simulink library "qss_tb_library_aalto"  (Simulink 8.3)
settings: Solver=ode45  SolverMode=SingleTasking  StartTime=0.0  StopTime=1220  RelTol=1e-3
undefined symbols (not defined in the file): c_BT_E1, c_BT_E2, c_BT_E3, c_BT_E4, c_BT_L1, c_BT_L2, c_BT_L3, c_BT_L4, cap_BT, cc_done, delta_h_C_air, DiscIntNeverNeededParam, dw_GG_c, eff_FC_max, eta_EG_map, eta_EM_map, g, h, H_o_m, H_u, I_BT_max, i_FC_in, i_FC_max, k1, k2, k3, k4, k_cs, M_air, manual_gearbox, P_CVT_opt, power_max, Q_BT_0, Q_BT_IC, Q_BT_min, Q_SC_IC, r_wheel, rchg_map_BT, rdis_map_BT, rho, rho_f, soc_map_BT, t_c, T_CE_max, T_EG_c, T_EG_max, T_EM_max, T_z, U_BT_0, V, V_CE_map, V_FC_out, voc_map_BT, w_CE_max, w_CE_upper, w_CVT_opt, w_EG_row, w_EG_upper, w_EM_row, w_EM_upper ... (+1)
libraries: simulink x4
(part 3 of 4)

== system qss_tb_library_aalto/Controller/Gen-set Controller/Engine start control ==
  speed (m/s) : Inport
  soc : Inport  Port=2
  Constant11 : Constant  Value=10  OutDataTypeStr=double
  Cst_Q_BT_max : Constant  Value=soc_max
  Cst_Q_BT_min : Constant  Value=soc_min
  Data Type Conversion2 : DataTypeConversion  OutDataTypeStr=double
  Engine on off : Subsystem
  Hit Crossing : HitCross  HitCrossingOffset=0.5  HitCrossingDirection=rising
  Logical operator1 : Logic  Operator=OR
  Logical operator2 : Logic  Operator=OR
  Logical operator3 : Logic  Operator=OR
  Relational Operator : RelationalOperator  Operator=<=  OutDataTypeStr=boolean
  Relational Operator1 : RelationalOperator  OutDataTypeStr=boolean
  Terminator2 : Terminator
  low speed : simulink/Logic and Bit Operations/Compare To Constant  relop=<=  const=1  OutDataTypeStr=boolean
  speed min-max : Relay  OnSwitchValue=spd_max/3.6  OffSwitchValue=spd_min/3.6  OutDataTypeStr=Inherit: Inherit via back propagation
  tempo : Subsystem
      mask Display: disp('Tempo')
  engine on : Outport
  wires:
  Cst_Q_BT_min/1 -> Relational Operator/2
  Relational Operator/1 -> Logical operator3/2
  Cst_Q_BT_max/1 -> Relational Operator1/2
  speed (m/s)/1 -> speed min-max/1, low speed/1
  Logical operator3/1 -> Engine on off/1(S)
  Logical operator1/1 -> Engine on off/2(R)
  Engine on off/2(!Q) -> Terminator2/1
  soc/1 -> Relational Operator/1, Relational Operator1/1
  Relational Operator1/1 -> Logical operator1/2
  Constant11/1 -> tempo/2(time)
  Hit Crossing/1 -> tempo/1(flag)
  Engine on off/1(Q) -> Data Type Conversion2/1
  Data Type Conversion2/1 -> Hit Crossing/1, Logical operator2/1
  tempo/1(tempo) -> Logical operator2/2
  Logical operator2/1 -> engine on/1
  low speed/1 -> Logical operator1/1
  speed min-max/1 -> Logical operator3/1

== system qss_tb_library_aalto/Controller/Gen-set Controller/Power control ==
  power (W) : Inport
  speed (m/s) : Inport  Port=2
  soc : Inport  Port=3
  engine on : Inport  Port=4
  Constant5 : Constant  Value=0  OutDataTypeStr=double
  Constant6 : Constant  Value=0  OutDataTypeStr=double
  Cst_ctrl_speed*pi_30 : Constant  Value=ctrl_speed*pi/30  OutDataTypeStr=double  SampleTime=Inf
  Engine off : Mux  Inputs=2
  Engine on : Mux  Inputs=2
  Sum1 : Sum  SaturateOnIntegerOverflow=on  InputSameDT=on  OutDataTypeStr=Inherit: Same as first input
  Sum2 : Sum  SaturateOnIntegerOverflow=on  InputSameDT=on  OutDataTypeStr=Inherit: Same as first input
  Switch1 : Switch  Criteria=u2 > Threshold  Threshold=0.5  SaturateOnIntegerOverflow=on  InputSameDT=on
  charging power : Lookup_n-D  NumberOfTableDimensions=1  BreakpointsForDimension1=[0 0.6 0.71 0.75 0.8 1]  Table=[power_max power_max 0 0 -power_max/2 -power_max/2]  RndMeth=Simplest  InputSameDT=on
  power limit : Saturate  UpperLimit=power_max  LowerLimit=0
  speed correction : Lookup_n-D  NumberOfTableDimensions=1  BreakpointsForDimension1=[0 120]/3.6  Table=[0 spd_coeff]  RndMeth=Simplest  InputSameDT=on
  torque : Product  Inputs=*/  SaturateOnIntegerOverflow=on  RndMeth=Zero  InputSameDT=on  OutDataTypeStr=Inherit: Same as first input
  ctrl cmds : Outport
  wires:
  Constant5/1 -> Engine off/1
  Constant6/1 -> Engine off/2
  Engine on/1 -> Switch1/1
  Engine off/1 -> Switch1/3
  Sum1/1 -> power limit/1
  power limit/1 -> torque/1
  torque/1 -> Engine on/2
  Cst_ctrl_speed*pi_30/1 -> Engine on/1, torque/2
  engine on/1 -> Switch1/2
  Switch1/1 -> ctrl cmds/1
  speed (m/s)/1 -> speed correction/1
  soc/1 -> Sum2/1
  Sum2/1 -> charging power/1
  charging power/1 -> Sum1/2
  power (W)/1 -> Sum1/1
  speed correction/1 -> Sum2/2

== system qss_tb_library_aalto/Driving Cycle/Driving Cycle/Differentiation ==
  V_z : Inport
  Sum1 : Sum  Inputs=+-  SaturateOnIntegerOverflow=on  InputSameDT=on  OutDataTypeStr=Inherit: Same as first input
  Unit Delay1 : UnitDelay  SampleTime=h
  D_z : Outport  InitialOutput=0
  wires:
  Unit Delay1/1 -> Sum1/2
  V_z/1 -> Sum1/1, Unit Delay1/1
  Sum1/1 -> D_z/1

== system qss_tb_library_aalto/Driving Cycle/Driving Cycle/Integration ==
  V_z : Inport
  Gain4 : Gain  Gain=0.5*h  SaturateOnIntegerOverflow=on  OutDataTypeStr=Inherit: Same as input  ParamDataTypeStr=Inherit: Same as input
  Plant : UnitDelay  InitialCondition=1  SampleTime=h
  Sum2 : Sum  SaturateOnIntegerOverflow=on  InputSameDT=on  OutDataTypeStr=Inherit: Same as first input
  Sum4 : Sum  SaturateOnIntegerOverflow=on  InputSameDT=on  OutDataTypeStr=Inherit: Same as first input
  Unit Delay2 : UnitDelay  SampleTime=h
  x_tot : Outport  InitialOutput=0
  wires:
  Sum2/1 -> Gain4/1
  Unit Delay2/1 -> Sum2/2
  V_z/1 -> Sum2/1, Unit Delay2/1
  Gain4/1 -> Sum4/2
  Sum4/1 -> Plant/1
  Plant/1 -> Sum4/1, x_tot/1

== system qss_tb_library_aalto/Driving Cycle/Driving Cycle v2/Differentiation ==
  V_z : Inport
  Sum1 : Sum  Inputs=+-  SaturateOnIntegerOverflow=on  InputSameDT=on  OutDataTypeStr=Inherit: Same as first input
  Unit Delay1 : UnitDelay  SampleTime=h
  D_z : Outport  InitialOutput=0
  wires:
  Sum1/1 -> D_z/1
  V_z/1 -> Unit Delay1/1, Sum1/1
  Unit Delay1/1 -> Sum1/2

== system qss_tb_library_aalto/Driving Cycle/Driving Cycle v2/Integration ==
  V_z : Inport
  Gain4 : Gain  Gain=0.5*h  SaturateOnIntegerOverflow=on  OutDataTypeStr=Inherit: Same as input  ParamDataTypeStr=Inherit: Same as input
  Plant : UnitDelay  InitialCondition=1  SampleTime=h
  Sum2 : Sum  SaturateOnIntegerOverflow=on  InputSameDT=on  OutDataTypeStr=Inherit: Same as first input
  Sum4 : Sum  SaturateOnIntegerOverflow=on  InputSameDT=on  OutDataTypeStr=Inherit: Same as first input
  Unit Delay2 : UnitDelay  SampleTime=h
  x_tot : Outport  InitialOutput=0
  wires:
  Plant/1 -> x_tot/1, Sum4/1
  Sum4/1 -> Plant/1
  Gain4/1 -> Sum4/2
  V_z/1 -> Unit Delay2/1, Sum2/1
  Unit Delay2/1 -> Sum2/2
  Sum2/1 -> Gain4/1

== system qss_tb_library_aalto/Driving Cycle/Driving Cycle v3/Differentiation ==
  V_z : Inport
  Sum1 : Sum  Inputs=+-  SaturateOnIntegerOverflow=on  InputSameDT=on  OutDataTypeStr=Inherit: Same as first input
  Unit Delay1 : UnitDelay  SampleTime=h
  D_z : Outport  InitialOutput=0
  wires:
  Unit Delay1/1 -> Sum1/2
  V_z/1 -> Sum1/1, Unit Delay1/1
  Sum1/1 -> D_z/1

== system qss_tb_library_aalto/Driving Cycle/Driving Cycle v3/Integration ==
  V_z : Inport
  Gain4 : Gain  Gain=0.5*h  SaturateOnIntegerOverflow=on  OutDataTypeStr=Inherit: Same as input  ParamDataTypeStr=Inherit: Same as input
  Plant : UnitDelay  InitialCondition=1  SampleTime=h
  Sum2 : Sum  SaturateOnIntegerOverflow=on  InputSameDT=on  OutDataTypeStr=Inherit: Same as first input
  Sum4 : Sum  SaturateOnIntegerOverflow=on  InputSameDT=on  OutDataTypeStr=Inherit: Same as first input
  Unit Delay2 : UnitDelay  SampleTime=h
  x_tot : Outport  InitialOutput=0
  wires:
  Sum2/1 -> Gain4/1
  Unit Delay2/1 -> Sum2/2
  V_z/1 -> Sum2/1, Unit Delay2/1
  Gain4/1 -> Sum4/2
  Sum4/1 -> Plant/1
  Plant/1 -> Sum4/1, x_tot/1

== system qss_tb_library_aalto/Energy Buffer/Battery/Battery voltage ==
  Q_BT : Inport
  P_BT : Inport  Port=2
  Charging : Subsystem
  Discharging : Subsystem
  Enable charging : Subsystem
  Enable discharging : Subsystem
  Enable idle : Subsystem
  Idle : Subsystem
  Product : Product  Inputs=/*  SaturateOnIntegerOverflow=on  RndMeth=Zero  InputSameDT=on  OutDataTypeStr=Inherit: Same as first input
  Supervision battery : Subsystem
  Switch : Switch  Threshold=0.5  SaturateOnIntegerOverflow=on  InputSameDT=on
  Switch1 : Switch  Threshold=0.5  SaturateOnIntegerOverflow=on  InputSameDT=on
  U_BT : Outport  InitialOutput=0
  I_BT : Outport  Port=2  InitialOutput=0
  wires:
  Enable idle/1(e_Z) -> Idle/Enable
  Charging/1(U_BT_L) -> Switch/1
  Switch1/1 -> Switch/3
  Idle/1(U_BT_E) -> Switch1/3
  Discharging/1(U_BT_E) -> Switch1/1
  P_BT/1 -> Charging/2(P_BT), Enable charging/1(P_BT), Enable idle/1(P_BT), Product/2, Discharging/2(P_BT), Enable discharging/1(P_BT)
  Enable discharging/1(e_E) -> Discharging/Enable, Switch1/2
  Product/1 -> Supervision battery/3(I_BT), I_BT/1
  Q_BT/1 -> Supervision battery/1(Q_BT), Charging/1(Q_BT), Discharging/1(Q_BT), Idle/1(Q_BT)
  Enable charging/1(e_E) -> Charging/Enable, Switch/2
  Switch/1 -> Product/1, Supervision battery/2(U_BT), U_BT/1

== system qss_tb_library_aalto/Energy Buffer/Battery v2/cell model ==
  current : Inport
  soc calculation : Subsystem
  voltage calculation : Subsystem
  voltage_out : Outport
  voc_out : Outport  Port=2
  rint_out : Outport  Port=3
  soc_out : Outport  Port=4
  wires:
  current/1 -> voltage calculation/2(Current), soc calculation/1(current)
  voltage calculation/3(Rint) -> rint_out/1
  voltage calculation/1(Voc) -> voc_out/1
  voltage calculation/2(voltage) -> voltage_out/1
  soc calculation/1(soc) -> voltage calculation/1(SOC (prev)), soc_out/1

== system qss_tb_library_aalto/Energy Buffer/Battery v3/cell model ==
  current : Inport
  Switch1 : Switch  SaturateOnIntegerOverflow=on  InputSameDT=on
  coulombic efficiency : Gain  Gain=0.99
  soc calculation : Subsystem
  voltage calculation : Subsystem
  voltage_out : Outport
  voc_out : Outport  Port=2
  rint_out : Outport  Port=3
  soc_out : Outport  Port=4
  wires:
  soc calculation/1(soc) -> soc_out/1, voltage calculation/1(SOC (prev))
  voltage calculation/2(voltage) -> voltage_out/1
  voltage calculation/1(Voc) -> voc_out/1
  voltage calculation/3(Rint) -> rint_out/1
  coulombic efficiency/1 -> Switch1/3
  current/1 -> coulombic efficiency/1, Switch1/1, Switch1/2
  Switch1/1 -> voltage calculation/2(Current), soc calculation/1(current)

== system qss_tb_library_aalto/Energy Buffer/Supercapacitor/Supervision supercap ==
  Q_SC : Inport
  P_SC : Inport  Port=2
  Charge: P > 0 : Gain  Gain=4*C_SC^2*R_SC  SaturateOnIntegerOverflow=on  OutDataTypeStr=Inherit: Same as input  ParamDataTypeStr=Inherit: Same as input
  Constant6 : Constant  Value=U_SC_max
  Constant7 : Constant  Value=P_SC_max
  Gain : Gain  Gain=1/C_SC  SaturateOnIntegerOverflow=on  OutDataTypeStr=Inherit: Same as input  ParamDataTypeStr=Inherit: Same as input
  Math Function : Math  Operator=square  SaturateOnIntegerOverflow=on
  Saturation1 : Saturate  UpperLimit=0  LowerLimit=-inf
  Saturation2 : Saturate  UpperLimit=0  LowerLimit=-inf
  Saturation3 : Saturate  UpperLimit=0  LowerLimit=-inf
  Stop Simulation : Stop
  Stop Simulation1 : Stop
  Stop Simulation2 : Stop
  Sum1 : Sum  Inputs=-+  SaturateOnIntegerOverflow=on  InputSameDT=on  OutDataTypeStr=Inherit: Same as first input
  Sum2 : Sum  Inputs=+-  SaturateOnIntegerOverflow=on  InputSameDT=on  OutDataTypeStr=Inherit: Same as first input
  Sum4 : Sum  SaturateOnIntegerOverflow=on  InputSameDT=on  OutDataTypeStr=Inherit: Same as first input
  wires:
  Math Function/1 -> Sum2/1
  Q_SC/1 -> Math Function/1, Gain/1
  Constant7/1 -> Sum4/2
  Constant6/1 -> Sum1/2
  Sum4/1 -> Saturation3/1
  Sum2/1 -> Saturation2/1
  Gain/1 -> Sum1/1
  Sum1/1 -> Saturation1/1
  Charge: P > 0/1 -> Sum2/2
  P_SC/1 -> Charge: P > 0/1, Sum4/1
  Saturation1/1 -> Stop Simulation/1
  Saturation2/1 -> Stop Simulation1/1
  Saturation3/1 -> Stop Simulation2/1

== system qss_tb_library_aalto/Energy Buffer/Supercapacitor v2/Supervision supercap ==
  Q_SC : Inport
  P_SC : Inport  Port=2
  Charge: P > 0 : Gain  Gain=4*C_SC^2*R_SC  SaturateOnIntegerOverflow=on  OutDataTypeStr=Inherit: Same as input  ParamDataTypeStr=Inherit: Same as input
  Constant6 : Constant  Value=U_SC_max
  Constant7 : Constant  Value=P_SC_max
  Gain : Gain  Gain=1/C_SC  SaturateOnIntegerOverflow=on  OutDataTypeStr=Inherit: Same as input  ParamDataTypeStr=Inherit: Same as input
  Math Function : Math  Operator=square  SaturateOnIntegerOverflow=on
  Saturation1 : Saturate  UpperLimit=0  LowerLimit=-inf
  Saturation2 : Saturate  UpperLimit=0  LowerLimit=-inf
  Saturation3 : Saturate  UpperLimit=0  LowerLimit=-inf
  Stop Simulation : Stop
  Stop Simulation1 : Stop
  Stop Simulation2 : Stop
  Sum1 : Sum  Inputs=-+  SaturateOnIntegerOverflow=on  InputSameDT=on  OutDataTypeStr=Inherit: Same as first input
  Sum2 : Sum  Inputs=+-  SaturateOnIntegerOverflow=on  InputSameDT=on  OutDataTypeStr=Inherit: Same as first input
  Sum4 : Sum  SaturateOnIntegerOverflow=on  InputSameDT=on  OutDataTypeStr=Inherit: Same as first input
  wires:
  Saturation3/1 -> Stop Simulation2/1
  Saturation2/1 -> Stop Simulation1/1
  Saturation1/1 -> Stop Simulation/1
  P_SC/1 -> Sum4/1, Charge: P > 0/1
  Charge: P > 0/1 -> Sum2/2
  Sum1/1 -> Saturation1/1
  Gain/1 -> Sum1/1
  Sum2/1 -> Saturation2/1
  Sum4/1 -> Saturation3/1
  Constant6/1 -> Sum1/2
  Constant7/1 -> Sum4/2
  Q_SC/1 -> Gain/1, Math Function/1
  Math Function/1 -> Sum2/1

== system qss_tb_library_aalto/Energy Buffer/Supercapacitor v3/Supervision supercap ==
  Q_SC : Inport
  P_SC : Inport  Port=2
  Charge: P > 0 : Gain  Gain=4*C_SC^2*R_SC  SaturateOnIntegerOverflow=on  OutDataTypeStr=Inherit: Same as input  ParamDataTypeStr=Inherit: Same as input
  Constant6 : Constant  Value=U_SC_max
  Constant7 : Constant  Value=P_SC_max
  Gain : Gain  Gain=1/C_SC  SaturateOnIntegerOverflow=on  OutDataTypeStr=Inherit: Same as input  ParamDataTypeStr=Inherit: Same as input
  Math Function : Math  Operator=square  SaturateOnIntegerOverflow=on
  Saturation1 : Saturate  UpperLimit=0  LowerLimit=-inf
  Saturation2 : Saturate  UpperLimit=0  LowerLimit=-inf
  Saturation3 : Saturate  UpperLimit=0  LowerLimit=-inf
  Stop Simulation : Stop
  Stop Simulation1 : Stop
  Stop Simulation2 : Stop
  Sum1 : Sum  Inputs=-+  SaturateOnIntegerOverflow=on  InputSameDT=on  OutDataTypeStr=Inherit: Same as first input
  Sum2 : Sum  Inputs=+-  SaturateOnIntegerOverflow=on  InputSameDT=on  OutDataTypeStr=Inherit: Same as first input
  Sum4 : Sum  SaturateOnIntegerOverflow=on  InputSameDT=on  OutDataTypeStr=Inherit: Same as first input
  wires:
  Math Function/1 -> Sum2/1
  Q_SC/1 -> Math Function/1, Gain/1
  Constant7/1 -> Sum4/2
  Constant6/1 -> Sum1/2
  Sum4/1 -> Saturation3/1
  Sum2/1 -> Saturation2/1
  Gain/1 -> Sum1/1
  Sum1/1 -> Saturation1/1
  Charge: P > 0/1 -> Sum2/2
  P_SC/1 -> Charge: P > 0/1, Sum4/1
  Saturation1/1 -> Stop Simulation/1
  Saturation2/1 -> Stop Simulation1/1
  Saturation3/1 -> Stop Simulation2/1

== system qss_tb_library_aalto/Energy Converter/Combustion Engine (Willans-approximation)/Detect fuel cutoff ==
  P_CE_fuel : Inport
  T_CE : Inport  Port=2
  Constant1 : Constant  Value=ENABLE_FUEL_CUTOFF
  Constant3 : Constant  Value=P_CE_cutoff
  Decision : Switch  Threshold=0.5
  Detect fuel cutoff : Switch  Threshold=T_CE_cutoff + 0.01  SaturateOnIntegerOverflow=on  InputSameDT=on
  P_CE : Outport
  wires:
  Decision/1 -> P_CE/1
  Constant1/1 -> Decision/2
  Detect fuel cutoff/1 -> Decision/1
  P_CE_fuel/1 -> Decision/3, Detect fuel cutoff/1
  T_CE/1 -> Detect fuel cutoff/2
  Constant3/1 -> Detect fuel cutoff/3

== system qss_tb_library_aalto/Energy Converter/Combustion Engine (Willans-approximation)/Detect idle ==
  P_CE_fuel : Inport
  w_CE : Inport  Port=2
  T_CE : Inport  Port=3
  Constant3 : Constant  Value=P_CE_idle
  Idle detection : Fcn  Expr=(u(1) <= w_CE_idle) * (u(2) <= T_CE_idle)
  Mux : Mux  Inputs=2
  Switch2 : Switch  Threshold=0.5  SaturateOnIntegerOverflow=on  InputSameDT=on
  P_CE : Outport  InitialOutput=0
  wires:
  Constant3/1 -> Switch2/1
  Switch2/1 -> P_CE/1
  P_CE_fuel/1 -> Switch2/3
  Idle detection/1 -> Switch2/2
  w_CE/1 -> Mux/1
  T_CE/1 -> Mux/2
  Mux/1 -> Idle detection/1

== system qss_tb_library_aalto/Energy Converter/Combustion Engine (Willans-approximation)/Engine efficiency ==
  w_CE : Inport
  T_CE : Inport  Port=2
  Constant3 : Constant  Value=p_me0g
  Product1 : Product  Inputs=*/  SaturateOnIntegerOverflow=on  RndMeth=Zero  InputSameDT=on  OutDataTypeStr=Inherit: Same as first input
  Sum : Sum  SaturateOnIntegerOverflow=on  InputSameDT=on  OutDataTypeStr=Inherit: Same as first input
  p_me : Fcn  Expr=4*pi*u/V_d
  p_me0 : Sum  SaturateOnIntegerOverflow=on  InputSameDT=on  OutDataTypeStr=Inherit: Same as first input
  p_mef : Fcn  Expr=k1 * (k2 + k3*(S^2)*(u^2)) * PI * sqrt(k4/B)
  p_mf : Fcn  Expr=u/e
  eta_CE : Outport  InitialOutput=0
  wires:
  Product1/1 -> eta_CE/1
  p_me/1 -> Sum/1, Product1/1
  Sum/1 -> p_mf/1
  p_mf/1 -> Product1/2
  p_me0/1 -> Sum/2
  T_CE/1 -> p_me/1
  w_CE/1 -> p_mef/1
  p_mef/1 -> p_me0/1
  Constant3/1 -> p_me0/2

== system qss_tb_library_aalto/Energy Converter/Combustion Engine (consumption map)/Detect fuel cutoff ==
  P_CE_fuel : Inport
  T_CE : Inport  Port=2
  Constant1 : Constant  Value=ENABLE_FUEL_CUTOFF
  Constant3 : Constant  Value=P_CE_cutoff
  Decision : Switch  Threshold=0.5
  Detect fuel cutoff : Switch  Threshold=T_CE_cutoff + 0.01  SaturateOnIntegerOverflow=on  InputSameDT=on
  P_CE : Outport
  wires:
  Constant3/1 -> Detect fuel cutoff/3
  T_CE/1 -> Detect fuel cutoff/2
  P_CE_fuel/1 -> Detect fuel cutoff/1, Decision/3
  Detect fuel cutoff/1 -> Decision/1
  Constant1/1 -> Decision/2
  Decision/1 -> P_CE/1

== system qss_tb_library_aalto/Energy Converter/Combustion Engine (consumption map)/Detect idle ==
  P_CE_fuel : Inport
  w_CE : Inport  Port=2
  T_CE : Inport  Port=3
  Constant3 : Constant  Value=P_CE_idle
  Idle detection : Fcn  Expr=(u(1) <= w_CE_idle) * (u(2) <= T_CE_idle)
  Mux : Mux  Inputs=2
  Switch2 : Switch  Threshold=0.5  SaturateOnIntegerOverflow=on  InputSameDT=on
  P_CE : Outport  InitialOutput=0
  wires:
  Mux/1 -> Idle detection/1
  T_CE/1 -> Mux/2
  w_CE/1 -> Mux/1
  Idle detection/1 -> Switch2/2
  P_CE_fuel/1 -> Switch2/3
  Switch2/1 -> P_CE/1
  Constant3/1 -> Switch2/1

== system qss_tb_library_aalto/Energy Converter/Combustion Engine (consumption map)/Detect overload and overspeed ==
  w_CE : Inport
  T_CE : Inport  Port=2
  Abs : Abs  SaturateOnIntegerOverflow=on
  Constant : Constant  Value=w_CE_upper
  Maximum torque : Lookup  InputValues=w_CE_max  Table=T_CE_max  SaturateOnIntegerOverflow=on
  Saturation : Saturate  UpperLimit=0  LowerLimit=-inf
  Saturation1 : Saturate  UpperLimit=0  LowerLimit=-inf
  Stop Simulation : Stop
  Stop Simulation1 : Stop
  Sum : Sum  Inputs=+-  SaturateOnIntegerOverflow=on  InputSameDT=on  OutDataTypeStr=Inherit: Same as first input
  Sum1 : Sum  Inputs=+-  SaturateOnIntegerOverflow=on  InputSameDT=on  OutDataTypeStr=Inherit: Same as first input
  wires:
  Sum/1 -> Saturation/1
  w_CE/1 -> Maximum torque/1, Sum1/2
  T_CE/1 -> Abs/1
  Maximum torque/1 -> Sum/1
  Abs/1 -> Sum/2
  Saturation/1 -> Stop Simulation/1
  Constant/1 -> Sum1/1
  Sum1/1 -> Saturation1/1
  Saturation1/1 -> Stop Simulation1/1

== system qss_tb_library_aalto/Energy Converter/Combustion Engine (hybrid vehicle)/Detect fuel cutoff ==
  P_CE_fuel : Inport
  T_CE : Inport  Port=2
  Constant1 : Constant  Value=ENABLE_FUEL_CUTOFF
  Constant3 : Constant  Value=P_CE_cutoff
  Decision : Switch  Threshold=0.5
  Detect fuel cutoff : Switch  Threshold=T_CE_cutoff + 0.01  SaturateOnIntegerOverflow=on  InputSameDT=on
  P_CE : Outport
  wires:
  Decision/1 -> P_CE/1
  Constant1/1 -> Decision/2
  Detect fuel cutoff/1 -> Decision/1
  P_CE_fuel/1 -> Decision/3, Detect fuel cutoff/1
  T_CE/1 -> Detect fuel cutoff/2
  Constant3/1 -> Detect fuel cutoff/3

== system qss_tb_library_aalto/Energy Converter/Combustion Engine (hybrid vehicle)/Detect idle ==
  P_CE_fuel : Inport
  w_CE : Inport  Port=2
  T_CE : Inport  Port=3
  Constant3 : Constant  Value=P_CE_idle
  Idle detection : Fcn  Expr=(u(1) <= w_CE_idle) * (u(2) <= T_CE_idle)
  Mux : Mux  Inputs=2
  Switch2 : Switch  Threshold=0.5  SaturateOnIntegerOverflow=on  InputSameDT=on
  P_CE : Outport  InitialOutput=0
  wires:
  Constant3/1 -> Switch2/1
  Switch2/1 -> P_CE/1
  P_CE_fuel/1 -> Switch2/3
  Idle detection/1 -> Switch2/2
  w_CE/1 -> Mux/1
  T_CE/1 -> Mux/2
  Mux/1 -> Idle detection/1

== system qss_tb_library_aalto/Energy Converter/Combustion Engine (hybrid vehicle)/Detect overload and overspeed ==
  w_CE : Inport
  T_CE : Inport  Port=2
  Abs : Abs  SaturateOnIntegerOverflow=on
  Constant : Constant  Value=w_CE_upper
  Maximum torque : Lookup  InputValues=w_CE_max  Table=T_CE_max  SaturateOnIntegerOverflow=on
  Saturation : Saturate  UpperLimit=0  LowerLimit=-inf
  Saturation1 : Saturate  UpperLimit=0  LowerLimit=-inf
  Stop Simulation : Stop
  Stop Simulation1 : Stop
  Sum : Sum  Inputs=+-  SaturateOnIntegerOverflow=on  InputSameDT=on  OutDataTypeStr=Inherit: Same as first input
  Sum1 : Sum  Inputs=+-  SaturateOnIntegerOverflow=on  InputSameDT=on  OutDataTypeStr=Inherit: Same as first input
  wires:
  Saturation1/1 -> Stop Simulation1/1
  Sum1/1 -> Saturation1/1
  Constant/1 -> Sum1/1
  Saturation/1 -> Stop Simulation/1
  Abs/1 -> Sum/2
  Maximum torque/1 -> Sum/1
  T_CE/1 -> Abs/1
  w_CE/1 -> Sum1/2, Maximum torque/1
  Sum/1 -> Saturation/1

== system qss_tb_library_aalto/Energy Converter/Combustion Engine (hybrid vehicle)/torque limit ==
  w : Inport
  T : Inport  Port=2
  Constant2 : Constant  Value=T_CE_cutoff
  Maximum torque : Lookup  InputValues=w_CE_max  Table=T_CE_max  SaturateOnIntegerOverflow=on
  saturation with inputs : Subsystem
  T_lim : Outport
  wires:
  Maximum torque/1 -> saturation with inputs/1(upper limit in)
  Constant2/1 -> saturation with inputs/3(lower limit in)
  w/1 -> Maximum torque/1
  T/1 -> saturation with inputs/2(signal in)
  saturation with inputs/1(signal out) -> T_lim/1

== system qss_tb_library_aalto/Energy Converter/Combustion Engine (hybrid vehicle) v2/Detect fuel cutoff ==
  P_CE_fuel : Inport
  T_ctrl : Inport  Port=2
  Constant1 : Constant  Value=ENABLE_FUEL_CUTOFF
  Constant3 : Constant  Value=P_CE_cutoff
  Decision : Switch  Threshold=0.5
  Detect fuel cutoff : Switch  SaturateOnIntegerOverflow=on  InputSameDT=on
  P_CE : Outport
  wires:
  Constant3/1 -> Detect fuel cutoff/3
  T_ctrl/1 -> Detect fuel cutoff/2
  P_CE_fuel/1 -> Detect fuel cutoff/1, Decision/3
  Detect fuel cutoff/1 -> Decision/1
  Constant1/1 -> Decision/2
  Decision/1 -> P_CE/1

== system qss_tb_library_aalto/Energy Converter/Combustion Engine (hybrid vehicle) v2/Detect idle ==
  w_CE : Inport
  T_in : Inport  Port=2
  Constant1 : Constant  Value=P_aux
  Constant11 : Constant  Value=0  OutDataTypeStr=double
  Constant2 : Constant  Value=w_CE_idle
  Constant3 : Constant  Value=P_CE_idle
  Idle detection : Fcn  Expr=(u(2) <= T_CE_idle)
  Mux : Mux  Inputs=2
  Power : Sum  SaturateOnIntegerOverflow=on  InputSameDT=on  OutDataTypeStr=Inherit: Same as first input
  Product : Product  SaturateOnIntegerOverflow=on  RndMeth=Zero  InputSameDT=on  OutDataTypeStr=Inherit: Same as first input
  Product1 : Product  Inputs=*/  SaturateOnIntegerOverflow=on  RndMeth=Zero  InputSameDT=on  OutDataTypeStr=Inherit: Same as first input
  Rate Limiter : RateLimiter  RisingSlewLimit=100  FallingSlewLimit=-250
  Switch1 : Switch  Criteria=u2 > Threshold  SaturateOnIntegerOverflow=on  InputSameDT=on
  Switch2 : Switch  Threshold=0.5  SaturateOnIntegerOverflow=on  InputSameDT=on
  Switch3 : Switch  Threshold=0.5  SaturateOnIntegerOverflow=on  InputSameDT=on
  w_out : Outport  InitialOutput=0
  T_out : Outport  Port=2  InitialOutput=0
  wires:
  Mux/1 -> Idle detection/1
  T_in/1 -> Product/1, Mux/2
  w_CE/1 -> Switch3/3, Product/2, Mux/1
  Idle detection/1 -> Switch3/2, Switch2/2
  Constant3/1 -> Switch2/1
  Constant1/1 -> Power/2
  Switch2/1 -> Power/1
  Product/1 -> Switch2/3
  Power/1 -> Product1/1
  Product1/1 -> Switch1/1
  Switch1/1 -> T_out/1
  Constant11/1 -> Switch1/3
  Constant2/1 -> Switch3/1
  Switch3/1 -> Rate Limiter/1
  Rate Limiter/1 -> Switch1/2, w_out/1, Product1/2

== system qss_tb_library_aalto/Energy Converter/Combustion Engine (hybrid vehicle) v2/Detect overload and overspeed ==
  w_CE : Inport
  T_CE : Inport  Port=2
  Abs : Abs  SaturateOnIntegerOverflow=on
  Constant : Constant  Value=w_CE_upper
  Maximum torque : Lookup  InputValues=w_CE_max  Table=T_CE_max  SaturateOnIntegerOverflow=on
  Saturation : Saturate  UpperLimit=0  LowerLimit=-inf
  Saturation1 : Saturate  UpperLimit=0  LowerLimit=-inf
  Stop Simulation : Stop
  Stop Simulation1 : Stop
  Sum : Sum  Inputs=+-  SaturateOnIntegerOverflow=on  InputSameDT=on  OutDataTypeStr=Inherit: Same as first input
  Sum1 : Sum  Inputs=+-  SaturateOnIntegerOverflow=on  InputSameDT=on  OutDataTypeStr=Inherit: Same as first input
  wires:
  Sum/1 -> Saturation/1
  w_CE/1 -> Maximum torque/1, Sum1/2
  T_CE/1 -> Abs/1
  Maximum torque/1 -> Sum/1
  Abs/1 -> Sum/2
  Saturation/1 -> Stop Simulation/1
  Constant/1 -> Sum1/1
  Sum1/1 -> Saturation1/1
  Saturation1/1 -> Stop Simulation1/1

== system qss_tb_library_aalto/Energy Converter/Combustion Engine (hybrid vehicle) v2/torque limit ==
  w : Inport
  T : Inport  Port=2
  Constant2 : Constant  Value=T_CE_cutoff
  Maximum torque : Lookup  InputValues=w_CE_max  Table=T_CE_max  SaturateOnIntegerOverflow=on
  saturation with inputs : Subsystem
  T_lim : Outport
  wires:
  saturation with inputs/1(signal out) -> T_lim/1
  T/1 -> saturation with inputs/2(signal in)
  w/1 -> Maximum torque/1
  Constant2/1 -> saturation with inputs/3(lower limit in)
  Maximum torque/1 -> saturation with inputs/1(upper limit in)

== system qss_tb_library_aalto/Energy Converter/Combustion Engine v2/Detect fuel cutoff ==
  P_CE_fuel : Inport
  T_CE : Inport  Port=2
  Constant1 : Constant  Value=ENABLE_FUEL_CUTOFF
  Constant3 : Constant  Value=P_CE_cutoff
  Decision : Switch  Threshold=0.5
  Detect fuel cutoff : Switch  Threshold=T_CE_cutoff + 0.01  SaturateOnIntegerOverflow=on  InputSameDT=on
  P_CE : Outport
  wires:
  Decision/1 -> P_CE/1
  Constant1/1 -> Decision/2
  Detect fuel cutoff/1 -> Decision/1
  P_CE_fuel/1 -> Decision/3, Detect fuel cutoff/1
  T_CE/1 -> Detect fuel cutoff/2
  Constant3/1 -> Detect fuel cutoff/3

== system qss_tb_library_aalto/Energy Converter/Combustion Engine v2/Detect idle ==
  P_CE_fuel : Inport
  w_CE : Inport  Port=2
  T_CE : Inport  Port=3
  Constant3 : Constant  Value=P_CE_idle
  Idle detection : Fcn  Expr=(u(1) <= w_CE_idle) * (u(2) <= T_CE_idle)
  Mux : Mux  Inputs=2
  Switch2 : Switch  Threshold=0.5  SaturateOnIntegerOverflow=on  InputSameDT=on
  P_CE : Outport  InitialOutput=0
  wires:
  Constant3/1 -> Switch2/1
  Switch2/1 -> P_CE/1
  P_CE_fuel/1 -> Switch2/3
  Idle detection/1 -> Switch2/2
  w_CE/1 -> Mux/1
  T_CE/1 -> Mux/2
  Mux/1 -> Idle detection/1

== system qss_tb_library_aalto/Energy Converter/Combustion Engine v2/Detect overload and overspeed ==
  w_CE : Inport
  T_CE : Inport  Port=2
  Abs : Abs  SaturateOnIntegerOverflow=on
  Constant : Constant  Value=w_CE_upper
  Maximum torque : Lookup  InputValues=w_CE_max  Table=T_CE_max  SaturateOnIntegerOverflow=on
  Saturation : Saturate  UpperLimit=0  LowerLimit=-inf
  Saturation1 : Saturate  UpperLimit=0  LowerLimit=-inf
  Stop Simulation : Stop
  Stop Simulation1 : Stop
  Sum : Sum  Inputs=+-  SaturateOnIntegerOverflow=on  InputSameDT=on  OutDataTypeStr=Inherit: Same as first input
  Sum1 : Sum  Inputs=+-  SaturateOnIntegerOverflow=on  InputSameDT=on  OutDataTypeStr=Inherit: Same as first input
  wires:
  Saturation1/1 -> Stop Simulation1/1
  Sum1/1 -> Saturation1/1
  Constant/1 -> Sum1/1
  Saturation/1 -> Stop Simulation/1
  Abs/1 -> Sum/2
  Maximum torque/1 -> Sum/1
  T_CE/1 -> Abs/1
  w_CE/1 -> Sum1/2, Maximum torque/1
  Sum/1 -> Saturation/1

== system qss_tb_library_aalto/Energy Converter/Combustion Engine v3/Detect fuel cutoff ==
  P_CE_fuel : Inport
  T_gear : Inport  Port=2
  Constant1 : Constant  Value=ENABLE_FUEL_CUTOFF
  Constant3 : Constant  Value=P_CE_cutoff
  Decision : Switch  Threshold=0.5
  Detect fuel cutoff : Switch  SaturateOnIntegerOverflow=on  InputSameDT=on
  P_CE : Outport
  wires:
  Constant3/1 -> Detect fuel cutoff/3
  T_gear/1 -> Detect fuel cutoff/2
  P_CE_fuel/1 -> Detect fuel cutoff/1, Decision/3
  Detect fuel cutoff/1 -> Decision/1
  Constant1/1 -> Decision/2
  Decision/1 -> P_CE/1

== system qss_tb_library_aalto/Energy Converter/Combustion Engine v3/Detect idle ==
  w_CE : Inport
  T_in : Inport  Port=2
  Constant1 : Constant  Value=P_aux
  Constant11 : Constant  Value=0  OutDataTypeStr=double
  Constant3 : Constant  Value=P_CE_idle
  Idle detection : Fcn  Expr=(u(1) <= w_CE_idle) * (u(2) <= T_CE_idle)
  Mux : Mux  Inputs=2
  Power : Sum  SaturateOnIntegerOverflow=on  InputSameDT=on  OutDataTypeStr=Inherit: Same as first input
  Product : Product  SaturateOnIntegerOverflow=on  RndMeth=Zero  InputSameDT=on  OutDataTypeStr=Inherit: Same as first input
  Product1 : Product  Inputs=*/  SaturateOnIntegerOverflow=on  RndMeth=Zero  InputSameDT=on  OutDataTypeStr=Inherit: Same as first input
  Switch1 : Switch  Criteria=u2 > Threshold  SaturateOnIntegerOverflow=on  InputSameDT=on
  Switch2 : Switch  Threshold=0.5  SaturateOnIntegerOverflow=on  InputSameDT=on
  T_out : Outport  InitialOutput=0
  wires:
  Mux/1 -> Idle detection/1
  T_in/1 -> Product/1, Mux/2
  w_CE/1 -> Switch1/2, Product1/2, Product/2, Mux/1
  Idle detection/1 -> Switch2/2
  Constant3/1 -> Switch2/1
  Constant1/1 -> Power/2
  Switch2/1 -> Power/1
  Product/1 -> Switch2/3
  Power/1 -> Product1/1
  Constant11/1 -> Switch1/3
  Product1/1 -> Switch1/1
  Switch1/1 -> T_out/1

== system qss_tb_library_aalto/Energy Converter/Combustion Engine v3/Detect overload and overspeed ==
  w_CE : Inport
  T_CE : Inport  Port=2
  Abs : Abs  SaturateOnIntegerOverflow=on
  Constant : Constant  Value=w_CE_upper
  Maximum torque : Lookup  InputValues=w_CE_max  Table=T_CE_max  SaturateOnIntegerOverflow=on
  Saturation : Saturate  UpperLimit=0  LowerLimit=-inf
  Saturation1 : Saturate  UpperLimit=0  LowerLimit=-inf
  Stop Simulation : Stop
  Stop Simulation1 : Stop
  Sum : Sum  Inputs=+-  SaturateOnIntegerOverflow=on  InputSameDT=on  OutDataTypeStr=Inherit: Same as first input
  Sum1 : Sum  Inputs=+-  SaturateOnIntegerOverflow=on  InputSameDT=on  OutDataTypeStr=Inherit: Same as first input
  wires:
  Sum/1 -> Saturation/1
  w_CE/1 -> Maximum torque/1, Sum1/2
  T_CE/1 -> Abs/1
  Maximum torque/1 -> Sum/1
  Abs/1 -> Sum/2
  Saturation/1 -> Stop Simulation/1
  Constant/1 -> Sum1/1
  Sum1/1 -> Saturation1/1
  Saturation1/1 -> Stop Simulation1/1

== system qss_tb_library_aalto/Energy Converter/Electric Generator/Detect overload and overspeed ==
  w_EG : Inport
  T_EG : Inport  Port=2
  Abs : Abs  SaturateOnIntegerOverflow=on
  Constant : Constant  Value=w_EG_upper
  Maximum torque : Lookup  InputValues=w_EG_row  Table=T_EG_max  SaturateOnIntegerOverflow=on
  Saturation : Saturate  UpperLimit=0  LowerLimit=-inf
  Saturation1 : Saturate  UpperLimit=0  LowerLimit=-inf
  Stop Simulation : Stop
  Stop Simulation1 : Stop
  Sum : Sum  Inputs=+-  SaturateOnIntegerOverflow=on  InputSameDT=on  OutDataTypeStr=Inherit: Same as first input
  Sum1 : Sum  Inputs=+-  SaturateOnIntegerOverflow=on  InputSameDT=on  OutDataTypeStr=Inherit: Same as first input
  wires:
  Sum/1 -> Saturation/1
  w_EG/1 -> Maximum torque/1, Sum1/2
  T_EG/1 -> Abs/1
  Maximum torque/1 -> Sum/1
  Abs/1 -> Sum/2
  Saturation/1 -> Stop Simulation/1
  Constant/1 -> Sum1/1
  Sum1/1 -> Saturation1/1
  Saturation1/1 -> Stop Simulation1/1

== system qss_tb_library_aalto/Energy Converter/Electric Generator v2/Detect overload and overspeed ==
  w_EG : Inport
  T_EG : Inport  Port=2
  Abs : Abs  SaturateOnIntegerOverflow=on
  Constant : Constant  Value=w_EG_upper
  Maximum torque : Lookup  InputValues=w_EG_row  Table=T_EG_max  SaturateOnIntegerOverflow=on
  Saturation : Saturate  UpperLimit=0  LowerLimit=-inf
  Saturation1 : Saturate  UpperLimit=0  LowerLimit=-inf
  Stop Simulation : Stop
  Stop Simulation1 : Stop
  Sum : Sum  Inputs=+-  SaturateOnIntegerOverflow=on  InputSameDT=on  OutDataTypeStr=Inherit: Same as first input
  Sum1 : Sum  Inputs=+-  SaturateOnIntegerOverflow=on  InputSameDT=on  OutDataTypeStr=Inherit: Same as first input
  wires:
  Saturation1/1 -> Stop Simulation1/1
  Sum1/1 -> Saturation1/1
  Constant/1 -> Sum1/1
  Saturation/1 -> Stop Simulation/1
  Abs/1 -> Sum/2
  Maximum torque/1 -> Sum/1
  T_EG/1 -> Abs/1
  w_EG/1 -> Sum1/2, Maximum torque/1
  Sum/1 -> Saturation/1

== system qss_tb_library_aalto/Energy Converter/Electric Generator v3/Detect overload and overspeed ==
  w_EG : Inport
  T_EG : Inport  Port=2
  Abs : Abs  SaturateOnIntegerOverflow=on
  Constant : Constant  Value=w_EG_upper
  Maximum torque : Lookup  InputValues=w_EG_row  Table=T_EG_max  SaturateOnIntegerOverflow=on
  Saturation : Saturate  UpperLimit=0  LowerLimit=-inf
  Saturation1 : Saturate  UpperLimit=0  LowerLimit=-inf
  Stop Simulation : Stop
  Stop Simulation1 : Stop
  Sum : Sum  Inputs=+-  SaturateOnIntegerOverflow=on  InputSameDT=on  OutDataTypeStr=Inherit: Same as first input
  Sum1 : Sum  Inputs=+-  SaturateOnIntegerOverflow=on  InputSameDT=on  OutDataTypeStr=Inherit: Same as first input
  wires:
  Saturation1/1 -> Stop Simulation1/1
  Sum1/1 -> Saturation1/1
  Constant/1 -> Sum1/1
  Saturation/1 -> Stop Simulation/1
  Abs/1 -> Sum/2
  Maximum torque/1 -> Sum/1
  T_EG/1 -> Abs/1
  w_EG/1 -> Sum1/2, Maximum torque/1
  Sum/1 -> Saturation/1

== system qss_tb_library_aalto/Energy Converter/Electric Motor/Detect overload and overspeed ==
  w_EM : Inport
  T_EM : Inport  Port=2
  Abs : Abs  SaturateOnIntegerOverflow=on
  Constant : Constant  Value=w_EM_upper
  Maximum torque : Lookup  InputValues=w_EM_row  Table=T_EM_max  SaturateOnIntegerOverflow=on
  Saturation : Saturate  UpperLimit=0  LowerLimit=-inf
  Saturation1 : Saturate  UpperLimit=0  LowerLimit=-inf
  Stop Simulation : Stop
  Stop Simulation1 : Stop
  Sum : Sum  Inputs=+-  SaturateOnIntegerOverflow=on  InputSameDT=on  OutDataTypeStr=Inherit: Same as first input
  Sum1 : Sum  Inputs=+-  SaturateOnIntegerOverflow=on  InputSameDT=on  OutDataTypeStr=Inherit: Same as first input
  wires:
  Saturation1/1 -> Stop Simulation1/1
  Sum1/1 -> Saturation1/1
  Constant/1 -> Sum1/1
  Saturation/1 -> Stop Simulation/1
  Abs/1 -> Sum/2
  Maximum torque/1 -> Sum/1
  T_EM/1 -> Abs/1
  w_EM/1 -> Sum1/2, Maximum torque/1
  Sum/1 -> Saturation/1

== system qss_tb_library_aalto/Energy Converter/Electric Motor v2/Detect overload and overspeed ==
  w_EM : Inport
  T_EM : Inport  Port=2
  Abs : Abs  SaturateOnIntegerOverflow=on
  Constant : Constant  Value=w_EM_upper
  Maximum torque : Lookup  InputValues=w_EM_row  Table=T_EM_max*over_factor  SaturateOnIntegerOverflow=on
  Saturation : Saturate  UpperLimit=0  LowerLimit=-inf
  Saturation1 : Saturate  UpperLimit=0  LowerLimit=-inf
  Stop Simulation : Stop
  Stop Simulation1 : Stop
  Sum : Sum  Inputs=+-  SaturateOnIntegerOverflow=on  InputSameDT=on  OutDataTypeStr=Inherit: Same as first input
  Sum1 : Sum  Inputs=+-  SaturateOnIntegerOverflow=on  InputSameDT=on  OutDataTypeStr=Inherit: Same as first input
  wires:
  Sum/1 -> Saturation/1
  w_EM/1 -> Maximum torque/1, Sum1/2
  T_EM/1 -> Abs/1
  Maximum torque/1 -> Sum/1
  Abs/1 -> Sum/2
  Saturation/1 -> Stop Simulation/1
  Constant/1 -> Sum1/1
  Sum1/1 -> Saturation1/1
  Saturation1/1 -> Stop Simulation1/1

== system qss_tb_library_aalto/Energy Converter/Fuel Cell/Compressor with E-motor ==
  note: Air mass flow
  P_FC : Inport
  1/2 O2 for 1 H2 : Gain  Gain=1/2  SaturateOnIntegerOverflow=on  OutDataTypeStr=Inherit: Same as input  ParamDataTypeStr=Inherit: Same as input
  Air enthalpy : Gain  Gain=delta_h_C_air  SaturateOnIntegerOverflow=on  OutDataTypeStr=Inherit: Same as input  ParamDataTypeStr=Inherit: Same as input
  Air to fuel ratio : Gain  Gain=l_air  SaturateOnIntegerOverflow=on  OutDataTypeStr=Inherit: Same as input  ParamDataTypeStr=Inherit: Same as input
  E-motor efficiency : Gain  Gain=1/eta_EM_C  SaturateOnIntegerOverflow=on  OutDataTypeStr=Inherit: Same as input  ParamDataTypeStr=Inherit: Same as input
  Inverse O2  fraction : Gain  Gain=100/21  SaturateOnIntegerOverflow=on  OutDataTypeStr=Inherit: Same as input  ParamDataTypeStr=Inherit: Same as input
  Lower heating value : Gain  Gain=1/H_o_m  SaturateOnIntegerOverflow=on  OutDataTypeStr=Inherit: Same as input  ParamDataTypeStr=Inherit: Same as input
  Molecular weight : Gain  Gain=M_air  SaturateOnIntegerOverflow=on  OutDataTypeStr=Inherit: Same as input  ParamDataTypeStr=Inherit: Same as input
  To Workspace4 : ToWorkspace  VariableName=P_EM_C  SampleTime=1
  Unit Delay : UnitDelay  SampleTime=h
  P_EM_C : Outport  InitialOutput=0
  wires:
  Air enthalpy/1 -> E-motor efficiency/1
  Air to fuel ratio/1 -> Air enthalpy/1
  Unit Delay/1 -> Lower heating value/1
  Molecular weight/1 -> Air to fuel ratio/1
  Lower heating value/1 -> 1/2 O2 for 1 H2/1
  1/2 O2 for 1 H2/1 -> Inverse O2  fraction/1
  Inverse O2  fraction/1 -> Molecular weight/1
  E-motor efficiency/1 -> P_EM_C/1, To Workspace4/1
  P_FC/1 -> Unit Delay/1

== system qss_tb_library_aalto/Energy Converter/Fuel Cell/Supervision of current density ==
  "   i_FC" : Inport
  Constant6 : Constant  Value=i_FC_max
  Saturation1 : Saturate  UpperLimit=0  LowerLimit=-inf
  Stop Simulation : Stop
  Sum1 : Sum  Inputs=+-  SaturateOnIntegerOverflow=on  InputSameDT=on  OutDataTypeStr=Inherit: Same as first input
  wires:
  "   i_FC"/1 -> Sum1/2
  Constant6/1 -> Sum1/1
  Sum1/1 -> Saturation1/1
  Saturation1/1 -> Stop Simulation/1

== system qss_tb_library_aalto/Energy Converter/Fuel Cell v2/Compressor with E-motor ==
  note: Air mass flow
  P_FC : Inport
  1/2 O2 for 1 H2 : Gain  Gain=1/2  SaturateOnIntegerOverflow=on  OutDataTypeStr=Inherit: Same as input  ParamDataTypeStr=Inherit: Same as input
  Air enthalpy : Gain  Gain=delta_h_C_air  SaturateOnIntegerOverflow=on  OutDataTypeStr=Inherit: Same as input  ParamDataTypeStr=Inherit: Same as input
  Air to fuel ratio : Gain  Gain=l_air  SaturateOnIntegerOverflow=on  OutDataTypeStr=Inherit: Same as input  ParamDataTypeStr=Inherit: Same as input
  E-motor efficiency : Gain  Gain=1/eta_EM_C  SaturateOnIntegerOverflow=on  OutDataTypeStr=Inherit: Same as input  ParamDataTypeStr=Inherit: Same as input
  Inverse O2  fraction : Gain  Gain=100/21  SaturateOnIntegerOverflow=on  OutDataTypeStr=Inherit: Same as input  ParamDataTypeStr=Inherit: Same as input
  Lower heating value : Gain  Gain=1/H_o_m  SaturateOnIntegerOverflow=on  OutDataTypeStr=Inherit: Same as input  ParamDataTypeStr=Inherit: Same as input
  Molecular weight : Gain  Gain=M_air  SaturateOnIntegerOverflow=on  OutDataTypeStr=Inherit: Same as input  ParamDataTypeStr=Inherit: Same as input
  To Workspace4 : ToWorkspace  VariableName=P_EM_C  SampleTime=1
  Unit Delay : UnitDelay  SampleTime=h
  P_EM_C : Outport  InitialOutput=0
  wires:
  Air enthalpy/1 -> E-motor efficiency/1
  Air to fuel ratio/1 -> Air enthalpy/1
  Unit Delay/1 -> Lower heating value/1
  Molecular weight/1 -> Air to fuel ratio/1
  Lower heating value/1 -> 1/2 O2 for 1 H2/1
  1/2 O2 for 1 H2/1 -> Inverse O2  fraction/1
  Inverse O2  fraction/1 -> Molecular weight/1
  E-motor efficiency/1 -> P_EM_C/1, To Workspace4/1
  P_FC/1 -> Unit Delay/1

== system qss_tb_library_aalto/Energy Converter/Fuel Cell v2/Limits ==
  crrnt : Inport
  eff : Inport  Port=2
  Constant1 : Constant  Value=eps
  eff max : Lookup  InputValues=i_FC_in  Table=eff_FC_max  SaturateOnIntegerOverflow=on
  limits : simulink/Discontinuities/Saturation Dynamic  OutMin=[]  OutMax=[]  OutDataTypeStr=Inherit: Same as second input  OutDataType=fixdt(1, 16)  OutScaling=2^-10  DoSatur=off
  eff_out : Outport
  wires:
  eff max/1 -> limits/1
  Constant1/1 -> limits/3
  crrnt/1 -> eff max/1
  eff/1 -> limits/2
  limits/1 -> eff_out/1

== system qss_tb_library_aalto/Energy Converter/Fuel Cell v2/Supervision of current density ==
  "   i_FC" : Inport
  Constant6 : Constant  Value=i_FC_max
  Saturation1 : Saturate  UpperLimit=0  LowerLimit=-inf
  Stop Simulation : Stop
  Sum1 : Sum  Inputs=+-  SaturateOnIntegerOverflow=on  InputSameDT=on  OutDataTypeStr=Inherit: Same as first input
  wires:
  "   i_FC"/1 -> Sum1/2
  Constant6/1 -> Sum1/1
  Sum1/1 -> Saturation1/1
  Saturation1/1 -> Stop Simulation/1

== system qss_tb_library_aalto/Energy Source/Hydrogen Tank/Integration ==
  P_fuel : Inport
  Constant : Constant  Value=1/H_u
  Constant1 : Constant  Value=1/42.7e6
  Fuel consumption : UnitDelay  SampleTime=h
  Fuel consumption1 : UnitDelay  SampleTime=h
  Gain1 : Gain  Gain=.5*h  SaturateOnIntegerOverflow=on  OutDataTypeStr=Inherit: Same as input  ParamDataTypeStr=Inherit: Same as input
  Gain3 : Gain  Gain=.5*h  SaturateOnIntegerOverflow=on  OutDataTypeStr=Inherit: Same as input  ParamDataTypeStr=Inherit: Same as input
  Product1 : Product  SaturateOnIntegerOverflow=on  RndMeth=Zero  InputSameDT=on  OutDataTypeStr=Inherit: Same as first input
  Product2 : Product  SaturateOnIntegerOverflow=on  RndMeth=Zero  InputSameDT=on  OutDataTypeStr=Inherit: Same as first input
  Sum{1..4} (4 alike) : Sum  SaturateOnIntegerOverflow=on  InputSameDT=on  OutDataTypeStr=Inherit: Same as first input
  To Workspace1 : ToWorkspace  VariableName=m_dot_fuel  SampleTime=-1
  To Workspace2 : ToWorkspace  VariableName=m_fuel  SampleTime=-1
  Unit Delay1 : UnitDelay  SampleTime=h
  Unit Delay3 : UnitDelay  SampleTime=h
  m_fuel : Outport  InitialOutput=0
  gas equivalent : Outport  Port=2  InitialOutput=0
  wires:
  Product2/1 -> To Workspace1/1, Sum4/2
  Sum4/1 -> Fuel consumption/1
  Fuel consumption/1 -> To Workspace2/1, Sum4/1, m_fuel/1
  Sum1/1 -> Gain3/1
  Unit Delay3/1 -> Sum1/2
  P_fuel/1 -> Sum2/1, Unit Delay1/1, Unit Delay3/1, Sum1/1
  Gain3/1 -> Product2/2
  Constant/1 -> Product2/1
  Sum2/1 -> Gain1/1
  Unit Delay1/1 -> Sum2/2
  Gain1/1 -> Product1/2
  Constant1/1 -> Product1/1
  Sum3/1 -> Fuel consumption1/1
  Fuel consumption1/1 -> gas equivalent/1, Sum3/1
  Product1/1 -> Sum3/2

== system qss_tb_library_aalto/Energy Source/Tank/Integration ==
  P_fuel : Inport
  Constant : Constant  Value=1/H_u
  Fuel consumption : UnitDelay  SampleTime=h
  Gain3 : Gain  Gain=.5*h  SaturateOnIntegerOverflow=on  OutDataTypeStr=Inherit: Same as input  ParamDataTypeStr=Inherit: Same as input
  Product2 : Product  SaturateOnIntegerOverflow=on  RndMeth=Zero  InputSameDT=on  OutDataTypeStr=Inherit: Same as first input
  Sum1 : Sum  SaturateOnIntegerOverflow=on  InputSameDT=on  OutDataTypeStr=Inherit: Same as first input
  Sum4 : Sum  SaturateOnIntegerOverflow=on  InputSameDT=on  OutDataTypeStr=Inherit: Same as first input
  To Workspace1 : ToWorkspace  VariableName=m_dot_fuel  SampleTime=-1
  To Workspace2 : ToWorkspace  VariableName=m_fuel  SampleTime=-1
  Unit Delay3 : UnitDelay  SampleTime=h
  m_fuel : Outport  InitialOutput=0
  wires:
  Constant/1 -> Product2/1
  Gain3/1 -> Product2/2
  P_fuel/1 -> Sum1/1, Unit Delay3/1
  Unit Delay3/1 -> Sum1/2
  Sum1/1 -> Gain3/1
  Fuel consumption/1 -> m_fuel/1, Sum4/1, To Workspace2/1
  Sum4/1 -> Fuel consumption/1
  Product2/1 -> Sum4/2, To Workspace1/1

== system qss_tb_library_aalto/Energy Source/Tank v2/Integration ==
  P_fuel : Inport
  Constant : Constant  Value=1/H_u
  Fuel consumption : UnitDelay  SampleTime=h
  Gain3 : Gain  Gain=.5*h  SaturateOnIntegerOverflow=on  OutDataTypeStr=Inherit: Same as input  ParamDataTypeStr=Inherit: Same as input
  Product2 : Product  SaturateOnIntegerOverflow=on  RndMeth=Zero  InputSameDT=on  OutDataTypeStr=Inherit: Same as first input
  Sum1 : Sum  SaturateOnIntegerOverflow=on  InputSameDT=on  OutDataTypeStr=Inherit: Same as first input
  Sum4 : Sum  SaturateOnIntegerOverflow=on  InputSameDT=on  OutDataTypeStr=Inherit: Same as first input
  To Workspace1 : ToWorkspace  VariableName=m_dot_fuel  SampleTime=-1
  To Workspace2 : ToWorkspace  VariableName=m_fuel  SampleTime=-1
  Unit Delay3 : UnitDelay  SampleTime=h
  m_fuel : Outport  InitialOutput=0
  wires:
  Product2/1 -> To Workspace1/1, Sum4/2
  Sum4/1 -> Fuel consumption/1
  Fuel consumption/1 -> To Workspace2/1, Sum4/1, m_fuel/1
  Sum1/1 -> Gain3/1
  Unit Delay3/1 -> Sum1/2
  P_fuel/1 -> Unit Delay3/1, Sum1/1
  Gain3/1 -> Product2/2
  Constant/1 -> Product2/1

== system qss_tb_library_aalto/Gear System/Continuously Variable Transmission/Power flow ==
  w_wheel : Inport
  T_wheel : Inport  Port=2
  j_CVT : Inport  Port=3
  "Engine -> Wheel" : Subsystem
  "Pwer Wheel -> Engine" : Subsystem
  Switch1 : Switch  SaturateOnIntegerOverflow=on  InputSameDT=on
  T_CVT : Outport  InitialOutput=0
  wires:
  "Pwer Wheel -> Engine"/1(T_CVT-) -> Switch1/3
  "Engine -> Wheel"/1(T_CVT+) -> Switch1/1
  Switch1/1 -> T_CVT/1
  j_CVT/1 -> "Engine -> Wheel"/3(j_CVT), "Pwer Wheel -> Engine"/3(j_CVT)
  w_wheel/1 -> "Pwer Wheel -> Engine"/1(w_wheel), "Engine -> Wheel"/1(w_wheel)
  T_wheel/1 -> "Pwer Wheel -> Engine"/2(T_wheel), "Engine -> Wheel"/2(T_wheel), Switch1/2

== system qss_tb_library_aalto/Gear System/Manual Gear Box/Power flow ==
  w_wheel : Inport
  T_wheel : Inport  Port=2
  gear : Inport  Port=3
  "Engine -> Wheel" : Subsystem
  Switch1 : Switch  SaturateOnIntegerOverflow=on  InputSameDT=on
  "Wheel -> Engine" : Subsystem
  T_MGB : Outport  InitialOutput=0
  wires:
  w_wheel/1 -> "Wheel -> Engine"/1(w_wheel), "Engine -> Wheel"/1(w_wheel)
  gear/1 -> "Wheel -> Engine"/3(gear), "Engine -> Wheel"/3(gear)
  "Wheel -> Engine"/1(T_MGB-) -> Switch1/3
  T_wheel/1 -> "Wheel -> Engine"/2(T_wheel), "Engine -> Wheel"/2(T_wheel), Switch1/2
  "Engine -> Wheel"/1(T_MGB+) -> Switch1/1
  Switch1/1 -> T_MGB/1

== system qss_tb_library_aalto/Gear System/Simple Transmission/Power flow ==
  w_wheel : Inport
  T_wheel : Inport  Port=2
  gear_ratio : Inport  Port=3
  "Energy Engine -> Wheel" : Subsystem
  "Energy Wheel -> Engine" : Subsystem
  Switch1 : Switch  SaturateOnIntegerOverflow=on  InputSameDT=on
  T_trans : Outport  InitialOutput=0
  wires:
  w_wheel/1 -> "Energy Wheel -> Engine"/1(w_wheel), "Energy Engine -> Wheel"/1(w_wheel)
  gear_ratio/1 -> "Energy Wheel -> Engine"/3(gear_ratio), "Energy Engine -> Wheel"/3(gear_ratio)
  "Energy Wheel -> Engine"/1(T_trans-) -> Switch1/3
  T_wheel/1 -> "Energy Wheel -> Engine"/2(T_wheel), "Energy Engine -> Wheel"/2(T_wheel), Switch1/2
  "Energy Engine -> Wheel"/1(T_trans+) -> Switch1/1
  Switch1/1 -> T_trans/1

== system qss_tb_library_aalto/Gear System/Transmission CE-EG/Power flow ==
  w_wheel : Inport
  T_wheel : Inport  Port=2
  gear_ratio : Inport  Port=3
  "Energy Engine -> Wheel" : Subsystem
  "Energy Wheel -> Engine" : Subsystem
  Switch1 : Switch  SaturateOnIntegerOverflow=on  InputSameDT=on
  T_trans : Outport  InitialOutput=0
  wires:
  Switch1/1 -> T_trans/1
  "Energy Engine -> Wheel"/1(T_trans+) -> Switch1/1
  T_wheel/1 -> Switch1/2, "Energy Engine -> Wheel"/2(T_wheel), "Energy Wheel -> Engine"/2(T_wheel)
  "Energy Wheel -> Engine"/1(T_trans-) -> Switch1/3
  gear_ratio/1 -> "Energy Engine -> Wheel"/3(gear_ratio), "Energy Wheel -> Engine"/3(gear_ratio)
  w_wheel/1 -> "Energy Engine -> Wheel"/1(w_wheel), "Energy Wheel -> Engine"/1(w_wheel)

== system qss_tb_library_aalto/Gear System/Transmission CE-EG v2/Power flow ==
  w_wheel : Inport
  T_wheel : Inport  Port=2
  gear_ratio : Inport  Port=3
  "Energy Engine -> Generator" : Subsystem
  "Energy Generator -> Engine" : Subsystem
  Switch1 : Switch  SaturateOnIntegerOverflow=on  InputSameDT=on
  T_trans : Outport  InitialOutput=0
  wires:
  w_wheel/1 -> "Energy Generator -> Engine"/1(w_wheel), "Energy Engine -> Generator"/1(w_wheel)
  gear_ratio/1 -> "Energy Generator -> Engine"/3(gear_ratio), "Energy Engine -> Generator"/3(gear_ratio)
  "Energy Generator -> Engine"/1(T_trans-) -> Switch1/3
  T_wheel/1 -> "Energy Generator -> Engine"/2(T_wheel), "Energy Engine -> Generator"/2(T_wheel), Switch1/2
  "Energy Engine -> Generator"/1(T_trans+) -> Switch1/1
  Switch1/1 -> T_trans/1

== system qss_tb_library_aalto/Gear System/Transmission Vehicle-EM/Power flow ==
  w_wheel : Inport
  T_wheel : Inport  Port=2
  gear_ratio : Inport  Port=3
  "Energy Engine -> Wheel" : Subsystem
  "Energy Wheel -> Engine" : Subsystem
  Switch1 : Switch  SaturateOnIntegerOverflow=on  InputSameDT=on
  T_trans : Outport  InitialOutput=0
  wires:
  Switch1/1 -> T_trans/1
  "Energy Engine -> Wheel"/1(T_trans+) -> Switch1/1
  T_wheel/1 -> Switch1/2, "Energy Engine -> Wheel"/2(T_wheel), "Energy Wheel -> Engine"/2(T_wheel)
  "Energy Wheel -> Engine"/1(T_trans-) -> Switch1/3
  gear_ratio/1 -> "Energy Engine -> Wheel"/3(gear_ratio), "Energy Wheel -> Engine"/3(gear_ratio)
  w_wheel/1 -> "Energy Engine -> Wheel"/1(w_wheel), "Energy Wheel -> Engine"/1(w_wheel)

== system qss_tb_library_aalto/Vehicle/Vehicle/Aerodynamic resistance ==
  v : Inport
  Aerodynamic resistance : Fcn  Expr=0.5*rho*cw*A_f*u^2
  To Workspace10 : ToWorkspace  VariableName=F_aero  SampleTime=-1
  F_aero : Outport  InitialOutput=0
  wires:
  v/1 -> Aerodynamic resistance/1
  Aerodynamic resistance/1 -> F_aero/1, To Workspace10/1

== system qss_tb_library_aalto/Vehicle/Vehicle/Average speed ==
  v : Inport
  Gain5 : Gain  Gain=0.5  SaturateOnIntegerOverflow=on  OutDataTypeStr=Inherit: Same as input  ParamDataTypeStr=Inherit: Same as input
  Sum2 : Sum  SaturateOnIntegerOverflow=on  InputSameDT=on  OutDataTypeStr=Inherit: Same as first input
  Unit Delay : UnitDelay  SampleTime=h
  v_a : Outport  InitialOutput=0
  wires:
  Unit Delay/1 -> Sum2/2
  Sum2/1 -> Gain5/1
  Gain5/1 -> v_a/1
  v/1 -> Sum2/1, Unit Delay/1

== system qss_tb_library_aalto/Vehicle/Vehicle/Inertia ==
  d_v : Inport
  Inertia : Fcn  Expr=m_f*(1+mt2m_f)*u/h
  To Workspace10 : ToWorkspace  VariableName=F_iner  SampleTime=-1
  F_iner : Outport  InitialOutput=0
  wires:
  Inertia/1 -> F_iner/1, To Workspace10/1
  d_v/1 -> Inertia/1
